simulink library "ChimeControlLibBtc"  (R2022b)
settings: Solver=VariableStepAuto  StartTime=0.0  StopTime=10.0  RelTol=1e-3
undefined symbols (not defined in the file or in its folder): chime_group_count, Row, spkrRouting
libraries: dspindex x10, RTC x3, FeaturePath x2, TOP x2, TuneVar x2, HandyTextFile x1
(part 2 of 2)

== matlab function ChimeControlLibBtc/ChimeControl/VolumeIndexToGainValue/Volume_Table_Translation ==
  data: scalarChimeControl_VolumeTable input; scalarChimeControl_Table_Idx output; scalarChimeControl_Table_dB output
  events: trigger input FUNCTION_CALL_EVENT
function [scalarChimeControl_Table_Idx,scalarChimeControl_Table_dB] = volume_table_translation(scalarChimeControl_VolumeTable)
%#codegen

% Set up the size and datatype of our TOP outputs:
maxTableSize = numel(scalarChimeControl_VolumeTable.Value) / 2;
idxType = 'uint8';
idxStorageType = 'uint32';
dbType = 'single';

% initialize table to zeros
scalarChimeControl_Table_Idx = zeros(1,maxTableSize,idxStorageType);
scalarChimeControl_Table_dB = zeros(1,maxTableSize,dbType);

% separate the pairs into their index and value components
givenPairs = scalarChimeControl_VolumeTable.Size(2);
indexes = scalarChimeControl_VolumeTable.Value(1,1:givenPairs);
values = scalarChimeControl_VolumeTable.Value(2,1:givenPairs);

% then sort and ignore duplicates
[cleanIdx,map] = unique(indexes);

% Validate input sizes
numPairs = numel(map);
argName='scalarChimeControl_VolumeTable';

% Validate: enough data?
if (numPairs < 2)
    TranslateError('%s must have at least 2 index pairs. Encounted value with only %f pairs\n', argName, numPairs);
end

% Validate: Highest index still below 1.0?
if (cleanIdx(end) > 1)
    TranslateError('%s out of range table index %f encountered. Index must be between 0 and 1.\n',argName,cleanIdx(end));
end

% fill in the table buffer with provided pairs
for i=1:numPairs
    scalarChimeControl_Table_Idx(i) = intmax(idxType) * cleanIdx(i);
    scalarChimeControl_Table_dB(i) = values(map(i));
end
% fill the rest of the table buffer with the last entry
for j=numel(map)+1:maxTableSize
    scalarChimeControl_Table_Idx(j) = scalarChimeControl_Table_Idx(numPairs);
    scalarChimeControl_Table_dB(j) =  scalarChimeControl_Table_dB(numPairs);
end


end

== matlab function ChimeControlLibBtc/ChimeControl/VolumeIndexToGainValue/calculate_vol_gain ==
  data: idx input; gain_value output; volTableIdx input; volTabledB input
function gain_value = Calculate_Vol_Table(idx, volTableIdx, volTabledB)
% gain_value = Calculate_Vol_Table(idx, volTableIdx, volTabledB)
%#codegen

iter=size(idx,2);
% initialize to zeros 
%gain_value = single(0.0);
gain_value=single(zeros(1,iter));
percent =zeros(1,iter);
lastIdx =zeros(1,iter);

for chind=1:iter
    j = uint8(1);
    % workaround to type problem
    idx(chind) = cast(idx(chind), class(volTableIdx(end)));
    
    %  bounds checking for vol - clip to max idx
    if (idx(chind) > volTableIdx(end))
        idx(chind) = volTableIdx(end);
    end
    
    % search through volume table to find index closest to vol
    while (j <= numel(volTableIdx))
        if (idx(chind) <= volTableIdx(j))
            if (j <= 1)
                % first indexed value is linearly interpolated to zero
                if (volTableIdx(j))
                    percent(chind) = single(idx(chind)) / single(volTableIdx(j));
                else
                    percent(chind) = single(1);
                end
                gain_value(chind) = percent(chind) * 10 ^ (volTabledB(j) / 20);
            else  
                % other values are interpolated in db space
                lastIdx(chind) = volTableIdx(j-1);
                percent(chind) = single(idx(chind) - lastIdx(chind)) / single(volTableIdx(j) - lastIdx(chind));
                gain_value(chind) = 10 ^ (((percent(chind) * (volTabledB(j) - volTabledB(j-1))) + volTabledB(j-1)) / 20);
            end
            break;
        else
            j = j + 1;
        end
    end
end

== matlab function ChimeControlLibBtc/ChimeControl/scalarchimeControl/Playback_Subsystemwith_StateMachine/playback_statemachine_function_singlechannel ==
  data: ch input; state input; playaback_flag input; countState input; countDecrement input; count input; forever input; y output; startOfFinalChime output; immediately input; chimeEndNotification input; endOfFinalChime input; startOfFinalChime input; CHECK_GROUP_COUNT input; CHIMECONTROL_NSTATES input; WAIT_FOR_PERIOD input; volume input; endOfFinalChime output; nextState_expired input; nextState_notExpired input; outputState input
function [y, startOfFinalChime, endOfFinalChime] = ...
    fcn(ch, state, playaback_flag, countState, countDecrement, count, forever, immediately, chimeEndNotification, endOfFinalChime, startOfFinalChime, CHECK_GROUP_COUNT, CHIMECONTROL_NSTATES, WAIT_FOR_PERIOD ,volume, nextState_expired, nextState_notExpired, outputState)

%WAIT_FOR_PERIOD=4;
nch=size(ch,2);
y=(zeros(1,nch));
IDLE = single(0);
RISE = single(1);
persistent state1;
persistent countState1;
persistent countDecrement1;
persistent count1;
persistent forever1;
persistent immediately1;
persistent state2;
persistent countState2;
persistent countDecrement2;
persistent count2;
persistent state_pre;
%persistent startOfFinalChime1;
%persistent endOfFinalChime1;
if(isempty(state1))
    state1 = state;
end
if(isempty(countState1))
    countState1 = countState;
end
if(isempty(countDecrement1))
    countDecrement1 = countDecrement;
end
if(isempty(count1))
    count1 = count;
end
if(isempty(forever1))
    forever1 = forever;
end
if(isempty(immediately1))
    immediately1 = immediately;
end
if(isempty(state_pre))
    state_pre = IDLE*single(ones(1,nch));
end

%% Call playback mode
for index=0:nch-1
    %% stop_playback call
    if (playaback_flag(index+1) == 0)
        [ state, countState1, countDecrement1,endOfFinalChime,startOfFinalChime]= stop_playback(index,immediately, state, countState1, countDecrement1, CHECK_GROUP_COUNT, CHIMECONTROL_NSTATES, chimeEndNotification, endOfFinalChime,startOfFinalChime);
    end
    
    %% start_playback call
    if (playaback_flag(index+1) == 1)
        [ state, countState1, countDecrement1,endOfFinalChime,startOfFinalChime] = start_playback(index,state, countState1, countDecrement1, forever, count, IDLE, RISE, CHECK_GROUP_COUNT, CHIMECONTROL_NSTATES,endOfFinalChime,startOfFinalChime);
    end
    
    %% testtone_playback call
    if (playaback_flag(index+1) == 2)
        [ state1,countState1,countDecrement1,endOfFinalChime,startOfFinalChime] = testtone_playback(index,state1,countState1,countDecrement1, CHIMECONTROL_NSTATES,endOfFinalChime,startOfFinalChime);
    end
    
end %% end of for loop for playback mode

% Main function is refactored to avoid warnings during MAB compliance
[y,state2,countState2,state_pre,countDecrement2,count2,startOfFinalChime, endOfFinalChime]= fcn1(y,nch,playaback_flag,IDLE,RISE,state2,countState2,countDecrement2,count2,state_pre,volume,state,count,countState1,countDecrement1,startOfFinalChime,endOfFinalChime,nextState_expired,nextState_notExpired,outputState,CHECK_GROUP_COUNT,CHIMECONTROL_NSTATES,WAIT_FOR_PERIOD);

end %% end of Main function

function [y,state2,countState2,state_pre,countDecrement2,count2,startOfFinalChime, endOfFinalChime]= fcn1(y,nch,playaback_flag,IDLE,RISE,state2,countState2,countDecrement2,count2,state_pre,volume,state,count,countState1,countDecrement1,startOfFinalChime,endOfFinalChime,nextState_expired,nextState_notExpired,outputState,CHECK_GROUP_COUNT,CHIMECONTROL_NSTATES,WAIT_FOR_PERIOD)
%% frameSize call
for index=0:nch-1
    if (playaback_flag(index+1) == 0)
        [state, countState1, countDecrement1, startOfFinalChime, endOfFinalChime] = state_machine(index,  state, count, countState1, countDecrement1, startOfFinalChime,endOfFinalChime, nextState_expired, nextState_notExpired, outputState, CHECK_GROUP_COUNT, CHIMECONTROL_NSTATES, WAIT_FOR_PERIOD);
        y(index+1) = volume(index+1)*(state(index+1)==RISE);
    end
    %% start_playback call
    if (playaback_flag(index+1) == 1)
        if(isempty(state2))
            state2 = state;
        end
        if(isempty(countState2))
            countState2 = countState1;
        end
        if(isempty(countDecrement2))
            countDecrement2 = countDecrement1;
        end
        if(isempty(count2))
            count2 = count;
        end
        % Condition check if count is set to 0 then current Chimes will play to finish without interruption.
        if( count(CHIMECONTROL_NSTATES*index+6)==0 && ...
                countState2(CHIMECONTROL_NSTATES*index+6)~=0 )
            count(CHIMECONTROL_NSTATES*index+6) = 1;
            countState2(CHIMECONTROL_NSTATES*index+6) = 1;
        end
        % this is the wake-up call to play Chimes per internal channel.
        if( state_pre(index+1)==IDLE && state(index+1)==RISE )
            state2(index+1)=state(index+1); 
            % hard coded constant 6 to avoid code gen complaining about dynamic array size.
            countState2(CHIMECONTROL_NSTATES*index+(1:6))=...
                countState1(CHIMECONTROL_NSTATES*index+(1:6));
            countDecrement2(CHIMECONTROL_NSTATES*index+(1:6))=...
                countDecrement1(CHIMECONTROL_NSTATES*index+(1:6));
            count2(CHIMECONTROL_NSTATES*index+(1:6))=...
                count(CHIMECONTROL_NSTATES*index+(1:6));
        end
        [state2, countState2, countDecrement2, startOfFinalChime, endOfFinalChime] = ...
            state_machine1(index,  state2, count, countState2, countDecrement2, ...
            startOfFinalChime,endOfFinalChime, nextState_expired, ...
            nextState_notExpired, outputState, CHECK_GROUP_COUNT, CHIMECONTROL_NSTATES, ...
            WAIT_FOR_PERIOD);
        % If RTC sents count 0, no output while traversing state machine.
        if( countState2(CHIMECONTROL_NSTATES*index+6)==0 )
            y(index+1) = volume(index+1)*0;
        % Normal operation in traversing state machine
        else
            y(index+1) = volume(index+1)*(state2(index+1)==RISE);
        end
    end
[y, state, state1, countState1, countDecrement1, startOfFinalChime, endOfFinalChime] = fcn2(y, state, RISE, volume, index, playaback_flag, state1, count, countState1, countDecrement1, startOfFinalChime,endOfFinalChime, nextState_expired, nextState_notExpired, outputState, CHECK_GROUP_COUNT, CHIMECONTROL_NSTATES, WAIT_FOR_PERIOD);
end %% end of for loop for playback mode
state_pre = state;
end %% End of fcn1 function

%% testtone_playback call
function [y, state, state1, countState1, countDecrement1, startOfFinalChime, endOfFinalChime] = fcn2(y, state, RISE, volume, index, playaback_flag, state1, count, countState1, countDecrement1, startOfFinalChime,endOfFinalChime, nextState_expired, nextState_notExpired, outputState, CHECK_GROUP_COUNT, CHIMECONTROL_NSTATES, WAIT_FOR_PERIOD)

    if (playaback_flag(index+1) == 2)
        [state1, countState1, countDecrement1, startOfFinalChime, endOfFinalChime] = state_machine(index,  state1, count, countState1, countDecrement1, startOfFinalChime,endOfFinalChime, nextState_expired, nextState_notExpired, outputState, CHECK_GROUP_COUNT, CHIMECONTROL_NSTATES, WAIT_FOR_PERIOD);
        y(index+1) = volume(index+1)*(state1(index+1)==RISE);
    end    
    if(state(index+1) == 0)
        state(index+1) = 0;
    elseif(state(index+1) == 1)
        state(index+1) = 1;
    end
end

%%% Stop playback function
function [state, countState1, countDecrement1, endOfFinalChime, startOfFinalChime] = stop_playback(ch,immediately, state, countState1, countDecrement1, CHECK_GROUP_COUNT, CHIMECONTROL_NSTATES, chimeEndNotification, endOfFinalChime,startOfFinalChime)

if( immediately(ch+1) )
    % Force idle state now
    state(ch+1) = 0;
    if (chimeEndNotification(ch+1))
        %endOfFinalChime(ch) = 1;
        endOfFinalChime(ch+1) = 1;
    end
else
    % Force last state's counter to 0
    idx = CHIMECONTROL_NSTATES*ch + CHECK_GROUP_COUNT;                        % idx is 0-based
    if (chimeEndNotification(ch+1))
        countState1(idx) = 1;        %% use "1" instead of "0", this would enable "endOfFinalChime" detection
    else
        countState1(idx) = 0;       %% use "0", this would disable "endOfFinalChime" detection.
    end
    
    %% Assign 0 for startOfFinalChime
    startOfFinalChime(ch+1) =0;
end

%% If chime is playing in forever mode, restore group countDecrement to 1
idx = (CHIMECONTROL_NSTATES*ch) + CHECK_GROUP_COUNT;
if(countDecrement1(idx) == 0 ) %% Indicates forever mode
    countDecrement1(idx) = 1;
end

end %%% End of stop_playback

%% start playback function
function [ state, countState1, countDecrement1, endOfFinalChime, startOfFinalChime] = start_playback(ch, state, countState1, countDecrement1, forever, count, IDLE, RISE, CHECK_GROUP_COUNT, CHIMECONTROL_NSTATES,endOfFinalChime,startOfFinalChime)

%  state(ch) = IDLE;
state(ch+1) = IDLE;

% Reset all counters for the channel

%   idx = CHIMECONTROL_NSTATES*ch + [0:CHIMECONTROL_NSTATES-1];   % idx is 0-based
%   countState(idx+1) = count(idx+1);
idx = CHIMECONTROL_NSTATES*ch ;   % idx is 0-based
for i=0:CHIMECONTROL_NSTATES-1
    idx=idx + 1;
    countState1(idx) = count(idx);
end

% If forever playback desired, set the last state's countDecrement to 0
% to prevent it from expiring
idx = CHIMECONTROL_NSTATES*ch + CHECK_GROUP_COUNT;              % idx is 0-based
if(forever(ch+1))
    countDecrement1(idx+1) = single(~forever(ch+1));
else
    countDecrement1(idx+1) = 1;
    %count(idx+1)=count(idx+1) - 1;
end
% Set rise/on state's countDecrement to 1 (in case it got overwritten by
% testtone_playback)
idx = CHIMECONTROL_NSTATES*ch + RISE;                        % idx is 0-based
countDecrement1(idx+1) = 1;

% Set state to chime rise/on
state(ch+1) = RISE;
%state(ch) = RISE;
%% Assign 1 for startOfFinalChime
startOfFinalChime(ch+1) =RISE;
%% Assign 0 for endOfFinalChime
endOfFinalChime(ch+1) = IDLE;
end %%% end of start_plyabck

%% testtone playback function
function [state1,countState1,countDecrement1, endOfFinalChime, startOfFinalChime] = testtone_playback(ch, state1,countState1,countDecrement1, CHIMECONTROL_NSTATES,endOfFinalChime,startOfFinalChime)
IDLE = 0;
RISE = 1;

% Go to idle state before we modify parameters (not really necessary for Matlab simulation)
%state(ch) = IDLE;
state1(ch+1) = IDLE;
% Set up rise/on state's counter to never expire so the machine will stay there forever
idx = CHIMECONTROL_NSTATES*ch + RISE;
countState1(idx+1) = 1;
countDecrement1(idx+1) = 0;
% Now go to rise/on state
%state(ch) = RISE;
state1(ch+1) = RISE;
%% Assign 1 for startOfFinalChime
startOfFinalChime(ch+1) =RISE;
%% Assign 0 for endOfFinalChime
endOfFinalChime(ch+1) = IDLE;
end %%% end of Testtone_plyaback

%% for stop and testtone statemachine
function [state1, countState1, countDecrement1, startOfFinalChime, endOfFinalChime] = state_machine(ch,  state1, count, countState1, countDecrement1, startOfFinalChime,endOfFinalChime, nextState_expired, nextState_notExpired, outputState, CHECK_GROUP_COUNT, CHIMECONTROL_NSTATES, WAIT_FOR_PERIOD)
% ch is 0-based
mstate1 = state1(ch+1);      % state is 0-based

% Run state machine
while(1)
    idx = CHIMECONTROL_NSTATES*ch + mstate1;        % idx is 0-based
    
    % Decrement state's counter
    countState1(idx+1) = countState1(idx+1) - countDecrement1(idx+1);
    countState_pre_update = countState1;
    
    % Counter expired?
    if( countState1(idx+1) <= 0 )
        % Yes
        countState1(idx+1) = count(idx+1);        % Reset counter
        mstate1 = nextState_expired(mstate1+1);
    else
        % No
        mstate1 = nextState_notExpired(mstate1+1);
    end
    
    % End this iteration of the state machine if we landed on an "output state"
    if( outputState(mstate1+1) )
        state1(ch+1) = mstate1;
        break;
    end
    
    %% Check if it's the start or end of the final chime
    idx = (CHIMECONTROL_NSTATES*ch);
    %% group count would be 2 just before the last chime starts
    if ( (state1(ch+1) == WAIT_FOR_PERIOD) && ( countState_pre_update(idx + WAIT_FOR_PERIOD) <= 1 ) && ( countState_pre_update(idx + CHECK_GROUP_COUNT) == 2 ) )
        startOfFinalChime(ch+1) = true;
    end
    %% group count would be 1 at (just before) the end of the last chime
    if ( (state1(ch+1) == WAIT_FOR_PERIOD) && ( countState_pre_update(idx + WAIT_FOR_PERIOD) <= 1 ) && ( countState_pre_update(idx + CHECK_GROUP_COUNT) == 1 ) )
        endOfFinalChime(ch+1) = true;
    end
end % state machine

end%% end of state_machinefunction
%% for start playback statemachine
function [state2, countState2, countDecrement2, startOfFinalChime, endOfFinalChime] = state_machine1(ch, state2, count, countState2, countDecrement2, startOfFinalChime,endOfFinalChime, nextState_expired, nextState_notExpired, outputState, CHECK_GROUP_COUNT, CHIMECONTROL_NSTATES, WAIT_FOR_PERIOD)
% ch is 0-based
mstate1 = state2(ch+1);      % state is 0-based

% Run state machine
while(1)
    idx = CHIMECONTROL_NSTATES*ch + mstate1;        % idx is 0-based
    
    % Decrement state's counter
    countState2(idx+1) = countState2(idx+1) - countDecrement2(idx+1);
    countState_pre_update = countState2;
    % Counter expired?
    if( countState2(idx+1) <= 0 )
        % Yes
        countState2(idx+1) = count(idx+1);        % Reset counter
        mstate1 = nextState_expired(mstate1+1);
    else
        % No
        mstate1 = nextState_notExpired(mstate1+1);
    end
    
    % End this iteration of the state machine if we landed on an "output state"
    if( outputState(mstate1+1) )
        state2(ch+1) = mstate1;
        break;
    end
    
    %% Check if it's the start or end of the final chime
    idx = (CHIMECONTROL_NSTATES*ch);
    %% group count would be 2 just before the last chime starts
    if ( (state2(ch+1) == WAIT_FOR_PERIOD) && ( countState_pre_update(idx + WAIT_FOR_PERIOD+1) <= 1 ) && ( countState_pre_update(idx + CHECK_GROUP_COUNT+1) == 2 ) )
        startOfFinalChime(ch+1) = true;
    end
    %% group count would be 1 at (just before) the end of the last chime
    if ( (state2(ch+1) == WAIT_FOR_PERIOD) && ( countState_pre_update(idx + WAIT_FOR_PERIOD+1) <= 1 ) && ( countState_pre_update(idx + CHECK_GROUP_COUNT+1) == 1 ) )
        endOfFinalChime(ch+1) = true;
    end
    
    
end % state machine

end%% end of state_machinefunction

== matlab function ChimeControlLibBtc/ChimeControl/MATLAB Function ==
  data: y output size=[1 nch]; nch parameter
function y = fcn(nch)
% alternative to using constant block
y = [1:1:nch];

== matlab function ChimeControlLibBtc/ChimeControl/scalarchimeControl/ChimeCancelSubsystem/If Action Subsystem/MATLAB Function ==
  data: y output size=[1 nch]; nch parameter
function y = fcn(nch)
% simple function to avoid using MATLAB experssion of BTC parameter in
% Constant block
y = single(ones(1,nch));

== matlab function ChimeControlLibBtc/ChimeControl/ChimeShapeConfiguration/Configurationfunction ==
  data: riseTime input; config_count1 output size=size(ones(1, nch*CHIMECONTROL_NSTATES)); onTime input; offTime input; numPulses input; period input; count input; Fs input; frameSize input
function config_count1  = fcn(riseTime, onTime, offTime, numPulses, period, count, Fs, frameSize)
 
 nch=length(riseTime);
 config_count1=single(zeros(1, nch*6));
 if any(offTime > max((period - (riseTime + onTime) .* numPulses), 0))     % off time needs to be restricted
      riseTime =single(zeros(nch,1)); onTime=single(zeros(nch,1));
  end
    
  onFrames           = round(Fs/frameSize.*(riseTime+onTime));
  periodDelayFrames  = round(Fs/frameSize.*offTime);
  periodFrames       = round(Fs/frameSize.*period);   

  offFrames          = round(Fs/frameSize.*((period - offTime)./numPulses - riseTime - onTime));    
  
  % additional checking for special cases  
  onFrames    = min(onFrames, periodFrames - 1);      % onFrames can be cut short by period
  offFrames   = max(offFrames, 1);                % offFrames >=0, just to be safe
  periodDelayFrames(onFrames == periodFrames - 1) = 0;     % no delay frames if rise time is cut short.

  config_count = [zeros(nch,1); onFrames; offFrames; numPulses; periodDelayFrames; count]; 
  config_count = reshape(config_count, size(ones(nch, 6)));
  %config_count = config_count(:)'; % Interleave to group a channels' parameters together
  k=0;
  for i=1:nch
      for j= 1:6
          k=k+1;
          config_count1(k)=config_count(i,j);
      end
  end
